simulink model "sltestTestSequenceWhenExample"  (R2017a)
settings: Solver=ode45  StartTime=0.0  StopTime=30.0  RelTol=1e-3  EnableMultiTasking=on
libraries: simulink x1
settings Model: Creator=The MathWorks, Inc.  LastModifiedBy=The MathWorks, Inc.
settings DataIOCC: LimitDataPoints=on  SaveFormat=Array
settings OptimizationCC: LifeSpan=inf
settings DebuggingCC: SolverPrmCheckMsg=warning  SFUnexpectedBacktrackingDiag=warning  SFNoUnconditionalDefaultTransitionDiag=warning  SFExecutionAtInitializationDiag=none
settings HardwareCC: ProdBitPerPointer=32  ProdBitPerSizeT=32  ProdBitPerPtrDiffT=32  ProdLargestAtomicFloat=None  ProdIntDivRoundTo=Undefined  ProdEndianess=Unspecified  ProdWordSize=32  ProdHWDeviceType=32-bit Generic
settings ModelReferenceCC: PropagateSignalLabelsOutOfModel=off
settings GRTTargetCC: TargetLangStandard=C89/C90 (ANSI)  GeneratePreprocessorConditionals=Disable all
settings ConfigComp: CovMetricSettings=dw  CovHtmlReporting=on  CovSaveCumulativeToWorkspaceVar=on  CovSaveSingleToWorkspaceVar=on  CovExternalEMLEnable=off  CovSFcnEnable=off

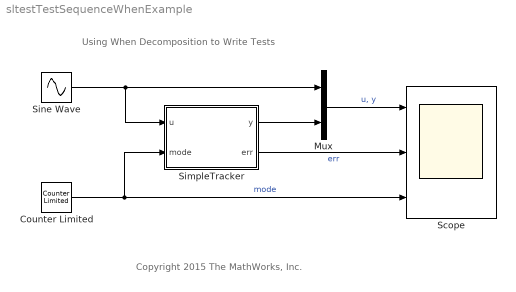
== system sltestTestSequenceWhenExample ==
  note: Using When Decomposition to Write Tests
  note: Copyright 2015 The MathWorks, Inc.
  Counter Limited : simulink/Sources/Counter Limited  uplimit=2  tsamp=10
  Mux : Mux  Inputs=2
  Scope : Scope  NumInputPorts=3
  SimpleTracker : Subsystem  TreatAsAtomicUnit=on  SystemSampleTime=0.1
  Sine Wave : Sin  Amplitude=5  SampleTime=0
  wires:
  Sine Wave/1 -> SimpleTracker/1(u), Mux/1
  Counter Limited/1 -> SimpleTracker/2(mode), Scope/3  "mode"
  SimpleTracker/1(y) -> Mux/2
  SimpleTracker/2(err) -> Scope/2  "err"
  Mux/1 -> Scope/1  "u, y"

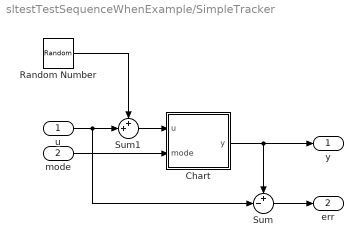
== system sltestTestSequenceWhenExample/SimpleTracker ==
  u : Inport
  mode : Inport  Port=2
  Chart : Stateflow chart  TreatAsAtomicUnit=on
  Random Number : RandomNumber  Variance=0.05  SampleTime=0.1
  Sum : Sum  Inputs=+-|
  Sum1 : Sum  Inputs=++|
  y : Outport
  err : Outport  Port=2
  wires:
  mode/1 -> Chart/2(mode)
  Chart/1(y) -> Sum/1, y/1
  u/1 -> Sum1/2, Sum/2
  Sum/1 -> err/1
  Sum1/1 -> Chart/1(u)
  Random Number/1 -> Sum1/1

== stateflow chart sltestTestSequenceWhenExample/SimpleTracker/Chart ==
  state TrackSlow
    en, du:
    y = y + 0.3 * (u - y);
  state TrackWait
  state TrackOff
    en:
    y = 0;
  state TrackQuick
    en, du:
    y = y + 0.7 * (u - y);
  TrackSlow -> TrackWait : [mode ~= 1]
  TrackWait -> TrackSlow [order 1] : after(0.4, sec)[mode == 1]
  TrackOff -> TrackWait : [mode ~= 0]
  (default) -> TrackOff
  TrackWait -> TrackOff [order 3] : after(0.4, sec)
  TrackQuick -> TrackWait : [mode ~= 2]
  TrackWait -> TrackQuick [order 2] : after(0.4, sec)[mode == 2]
  data: y output; u input; mode input
